simulink model "model"  (R2020b)
settings: Solver=FixedStepAuto  StartTime=0.0  StopTime=9  FixedStep=0.01  RelTol=1e-3
settings Model: Creator=Arvind Hishikar  LastModifiedBy=Arvind Hishikar

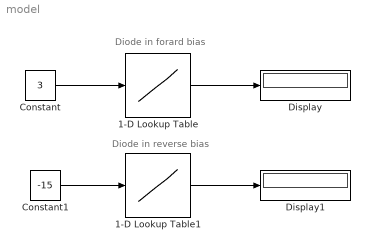
== system model ==
  note: Diode in reverse bias
  note: Diode in forard bias
  1-D Lookup Table : Lookup_n-D  NumberOfTableDimensions=1  BreakpointsForDimension1=[0 0.2 0.4 0.8 1.2 1.6 1.8 2.0 2.2 2.4]  BreakpointsForDimension10FirstPoint=-0.9360968731195527  Table=[ 0 0 0.5 2 5 10 15 20 25 30]  InternalRulePriority=Speed  RndMeth=Simplest  InputSameDT=on
  1-D Lookup Table1 : Lookup_n-D  NumberOfTableDimensions=1  BreakpointsForDimension1=[-25 -23 -21 -19 -17 -15 -11 -9 -7 -5 0]  Table=[25 15 13 11 9 7 4 3 2 1 0]  InternalRulePriority=Speed  RndMeth=Simplest  InputSameDT=on
  Constant : Constant  Value=3
  Constant1 : Constant  Value=-15
  Display : Display
  Display1 : Display
  wires:
  Constant/1 -> 1-D Lookup Table/1
  1-D Lookup Table/1 -> Display/1
  Constant1/1 -> 1-D Lookup Table1/1
  1-D Lookup Table1/1 -> Display1/1
